simulink model "vitesse"  (R2020a)
settings: Solver=VariableStepAuto  StartTime=0.0  StopTime=0.05  RelTol=1e-3
values from neighbouring files (symbols this model uses):
  Kb = (7.1875/0.5)/(0.233)    (= 61.69527897)    [be_trot.m]
  Tc2 = 1.592e-2    (= 0.01592)    [be_trot.m]
  Ti2 = 3.606e-3    (= 0.003606)    [be_trot.m]
settings Model: Creator=lagrost  LastModifiedBy=lagrost

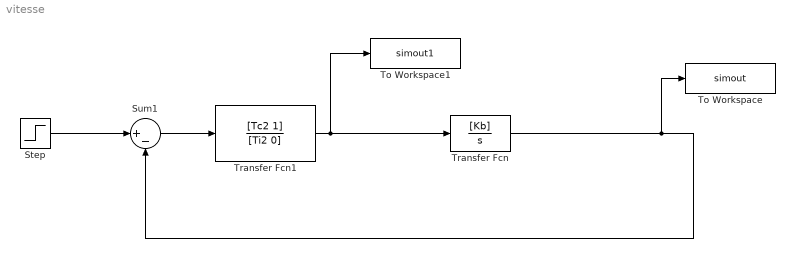
== system vitesse ==
  Step : Step  Time=0  After=0.233  SampleTime=0
  Sum1 : Sum  Inputs=|+-
  To Workspace : ToWorkspace  VariableName=simout  SaveFormat=Timeseries  SampleTime=-1
  To Workspace1 : ToWorkspace  VariableName=simout1  SaveFormat=Timeseries  SampleTime=-1
  Transfer Fcn : TransferFcn  Numerator=[Kb]  Denominator=[1 0]
  Transfer Fcn1 : TransferFcn  Numerator=[Tc2 1]  Denominator=[Ti2 0]
  wires:
  Step/1 -> Sum1/1
  Sum1/1 -> Transfer Fcn1/1
  Transfer Fcn/1 -> Sum1/2, To Workspace/1
  Transfer Fcn1/1 -> Transfer Fcn/1, To Workspace1/1
